simulink model "nmpc_sim"  (R2022a)
settings: Solver=ode45  StartTime=0.0  StopTime=10  RelTol=1e-3
values from neighbouring files (symbols this model uses):
  D = MassM(sr_info, q, A)    [sr_state_func.m]
libraries: mpclib x1
settings Model: Creator=charl  LastModifiedBy=charl

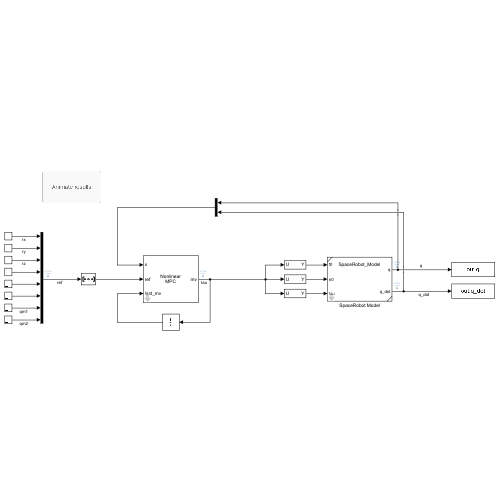
[thumbnail: Simulink's stored preview of the top-level diagram]
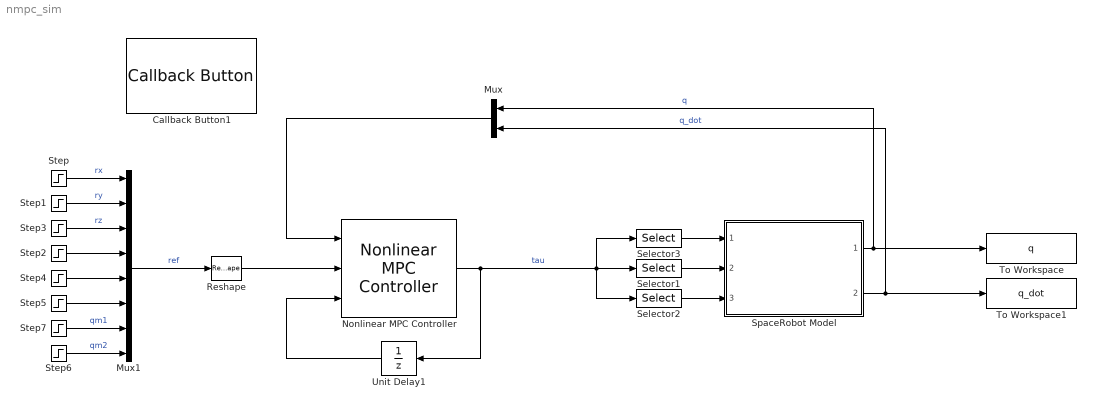
== system nmpc_sim ==
  Callback Button1 : CallbackButton  ButtonText=Animate results
      settings: ClickFcn=|
      | close all
      | try
      |     sr.animate(out.q, 'fps', 17, 'rate', 1);
      | catch
      |     close all
      | end
  Mux : Mux  Inputs=2
  Mux1 : Mux  Inputs=8
  Nonlinear MPC Controller : mpclib/Nonlinear MPC Controller  SCDEnableBlockLinearizationSpecification=on  nlmpcobj=nlobj  UseObjectTs=on  UseMEX=off  md_enabled=off  mvtarget_enabled=off  param_enabled=off  cost_enabled=off  mvseq_enabled=off  stateseq_enabled=off  ovseq_enabled=off  slack_enabled=off  status_enabled=off  ov_min=off  ov_max=off  mv_min=off  mv_max=off  mvrate_min=off  mvrate_max=off  state_min=off  state_max=off  ov_weight=off  mv_weight=off  mvrate_weight=off  ecr_weight=off  nlp_initialize=off
  Reshape : Reshape  OutputDimensionality=Row vector (2-D)
  Selector1 : Selector  IndexOptions=Index vector (dialog)  Indices=[4:6]  OutputSizes=1
  Selector2 : Selector  IndexOptions=Index vector (dialog)  Indices=[7:8]  OutputSizes=1
  Selector3 : Selector  IndexOptions=Index vector (dialog)  Indices=[1:3]  OutputSizes=1
  SpaceRobot Model : Subsystem  ReferencedSubsystem=SpaceRobot_Model  q_0=zeros(8, 1)  q_dot_0=zeros(8, 1)  spaceRobot=sr
  Step : Step  Time=0.1  After=0.5  SampleTime=0
  Step1 : Step  Time=2  After=0.5  SampleTime=0
  Step{2..6} (5 alike) : Step  After=0  SampleTime=0
  Step7 : Step  Time=5  After=pi/4  SampleTime=0
  To Workspace : ToWorkspace  VariableName=q  SaveFormat=Timeseries  SampleTime=-1
  To Workspace1 : ToWorkspace  VariableName=q_dot  SaveFormat=Timeseries  SampleTime=-1
  Unit Delay1 : UnitDelay  SampleTime=-1  HasFrameUpgradeWarning=on
  wires:
  Nonlinear MPC Controller/1 -> Selector3/1, Selector2/1, Selector1/1, Unit Delay1/1  "tau"
  Selector2/1 -> SpaceRobot Model/3
  Selector1/1 -> SpaceRobot Model/2
  Selector3/1 -> SpaceRobot Model/1
  Unit Delay1/1 -> Nonlinear MPC Controller/3
  Mux1/1 -> Reshape/1  "ref"
  Reshape/1 -> Nonlinear MPC Controller/2
  SpaceRobot Model/2 -> To Workspace1/1, Mux/2  "q_dot"
  SpaceRobot Model/1 -> To Workspace/1, Mux/1  "q"
  Step/1 -> Mux1/1  "rx"
  Step1/1 -> Mux1/2  "ry"
  Step3/1 -> Mux1/3  "rz"
  Step2/1 -> Mux1/4
  Step4/1 -> Mux1/5
  Step6/1 -> Mux1/8  "qm2"
  Step7/1 -> Mux1/7  "qm1"
  Step5/1 -> Mux1/6
  Mux/1 -> Nonlinear MPC Controller/1
